simulink model "nav21"  (R2020a)
settings: Solver=FixedStepDiscrete  StartTime=0.0  StopTime=inf  RelTol=1e-3
model workspace (MAT data in the model file):
  SL_ROS_VariableLengthArrays_MaxSizes.CommonInfo.ArrayTruncateAction = 'EmitWarning'
  SL_ROS_VariableLengthArrays_MaxSizes.MsgTypeMap = containers.Map
  SL_ROS_VariableLengthArrays_MaxSizes.MsgTypeMap.serialization.keys = {'nav_msgs/OccupancyGrid', 'sensor_msgs/CompressedImage', 'sensor_msgs/Image', 'std_msgs/Float64MultiArray'}
  SL_ROS_VariableLengthArrays_MaxSizes.MsgTypeMap.serialization.values{1}.PropertyName = 'Data'
  SL_ROS_VariableLengthArrays_MaxSizes.MsgTypeMap.serialization.values{1}.DataType = 'int8'
  SL_ROS_VariableLengthArrays_MaxSizes.MsgTypeMap.serialization.values{1}.MaxLength = 1000000
  SL_ROS_VariableLengthArrays_MaxSizes.MsgTypeMap.serialization.values{2}(1).PropertyName = 'Data'
  SL_ROS_VariableLengthArrays_MaxSizes.MsgTypeMap.serialization.values{2}(1).DataType = 'uint8'
  SL_ROS_VariableLengthArrays_MaxSizes.MsgTypeMap.serialization.values{2}(1).MaxLength = 36000
  SL_ROS_VariableLengthArrays_MaxSizes.MsgTypeMap.serialization.values{2}(2).PropertyName = 'Format'
  SL_ROS_VariableLengthArrays_MaxSizes.MsgTypeMap.serialization.values{2}(2).DataType = 'uint8'
  SL_ROS_VariableLengthArrays_MaxSizes.MsgTypeMap.serialization.values{2}(2).MaxLength = 128
  SL_ROS_VariableLengthArrays_MaxSizes.MsgTypeMap.serialization.values{3}(1).PropertyName = 'Data'
  SL_ROS_VariableLengthArrays_MaxSizes.MsgTypeMap.serialization.values{3}(1).DataType = 'uint8'
  SL_ROS_VariableLengthArrays_MaxSizes.MsgTypeMap.serialization.values{3}(1).MaxLength = 921600
  SL_ROS_VariableLengthArrays_MaxSizes.MsgTypeMap.serialization.values{3}(2).PropertyName = 'Encoding'
  SL_ROS_VariableLengthArrays_MaxSizes.MsgTypeMap.serialization.values{3}(2).DataType = 'uint8'
  SL_ROS_VariableLengthArrays_MaxSizes.MsgTypeMap.serialization.values{3}(2).MaxLength = 128
  SL_ROS_VariableLengthArrays_MaxSizes.MsgTypeMap.serialization.values{4}.PropertyName = 'Data'
  SL_ROS_VariableLengthArrays_MaxSizes.MsgTypeMap.serialization.values{4}.DataType = 'double'
  SL_ROS_VariableLengthArrays_MaxSizes.MsgTypeMap.serialization.values{4}.MaxLength = 32
  SL_ROS_VariableLengthArrays_MaxSizes.MsgTypeMap.serialization.uniformity = 0
  SL_ROS_VariableLengthArrays_MaxSizes.MsgTypeMap.serialization.keyType = 'char'
  SL_ROS_VariableLengthArrays_MaxSizes.MsgTypeMap.serialization.valueType = 'any'
values from neighbouring files (symbols this model uses):
  chargingStn = [setInitialPose(1,1), setInitialPose(1,2)]    [startup.m]
  L2RTransform = [cos(L2Rtheta), -sin(L2Rtheta), L2Rx ... (first row only)    [startup.m]
  LIVE_MODE = 1    [startup.m]
  map = binaryOccupancyMap(logicalMap, 1/0.05)    [exampleHelperVisualizeExecuteRobots.m]
  W2LOTransform = W2ORTransform/(L2RTransform)    [startup.m]
  W2ORtheta = setInitialPose(1,3)    [startup.m]
  waypoints = [-2.5, 0 ... (first row only)    [startup.m]
  wheelBase = 0.4464    [startup.m]
  wheelRadius = 0.1715/2    (= 0.08575)    [startup.m]
undefined symbols (not defined in the file or in its folder): Angular, Data, Data_SL_Info, gray, Linear, loadingStn, unloadingStn
libraries: robotlib x14, robotalgslib x3, simulink x2, vrlib x1
settings Model: EnablePacing=on  OrderedModelArguments=off  Creator=john  LastModifiedBy=john
settings OptimizationCC: EnhancedBackFolding=on  PassReuseOutputArgsAs=Individual arguments  ZeroExternalMemoryAtStartup=off  ZeroInternalMemoryAtStartup=off  MaxStackSize=64  OptimizeBlockOrder=speed  DifferentSizesBufferReuse=on  OptimizationCustomize=off  EfficientTunableParamExpr=on
settings DebuggingCC: ParameterTunabilityLossMsg=error
settings HardwareCC: ProdBitPerPointer=32  ProdBitPerSizeT=32  ProdBitPerPtrDiffT=32  ProdLargestAtomicFloat=None  ProdIntDivRoundTo=Undefined  ProdEndianess=Unspecified  ProdWordSize=32  ProdHWDeviceType=Generic->Unspecified (assume 32-bit Generic)  UseEmbeddedCoderFeatures=off
settings RTWCC: SystemTargetFile=ert.tlc  HardwareBoard=Robot Operating System (ROS)  TemplateMakefile=ert_default_tmf  Toolchain=Catkin  TargetLang=C++
settings CodeAppCC: ForceParamTrailComments=on  IgnoreCustomStorageClasses=off  OperatorAnnotations=on  SimulinkDataObjDesc=on  SFDataObjDesc=on  InsertBlockDesc=on
settings ERTTargetCC: SupportNonInlinedSFcns=on

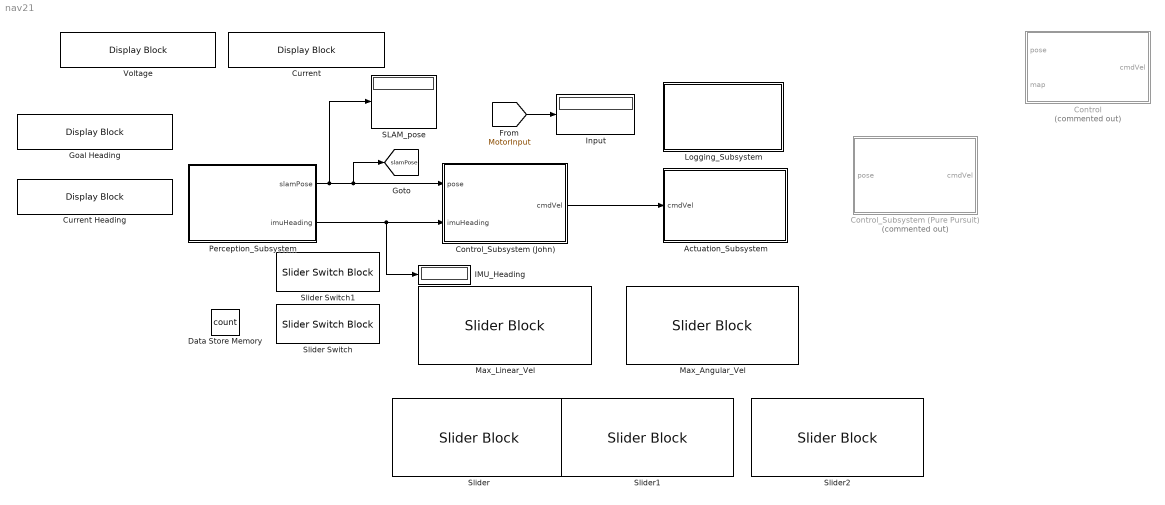
== system nav21 ==
  Actuation_Subsystem : Subsystem
  Control : Subsystem  Commented=on
  Control_Subsystem (John) : Subsystem
  Control_Subsystem (Pure Pursuit) : Subsystem  Commented=on
  Current : DisplayBlock  LabelPosition=Hide  Format=short  Transparency=1
  Current Heading : DisplayBlock  LabelPosition=Hide  Format=short  Transparency=1
  Data Store Memory : DataStoreMemory  DataStoreName=count  ReadBeforeWriteMsg=warning  WriteAfterWriteMsg=warning  WriteAfterReadMsg=warning  ShowAdditionalParam=off
  Goal Heading : DisplayBlock  LabelPosition=Hide  Format=short  Transparency=1
  IMU_Heading : Display
  Input : Display
  Logging_Subsystem : Subsystem
  Max_Angular_Vel : SliderBlock  ScaleMax=2
  Max_Linear_Vel : SliderBlock  ScaleMax=1.5
  Perception_Subsystem : Subsystem
  SLAM_pose : Display
  Slider : SliderBlock  ScaleMax=5
  Slider Switch : SliderSwitchBlock
      settings: Values={{'Off', 'On'}, [0 1]}
  Slider Switch1 : SliderSwitchBlock
      settings: Values={{'Off', 'On'}, [1 0]}
  Slider1 : SliderBlock  ScaleMax=1
  Slider2 : SliderBlock  ScaleMax=1.5
  Voltage : DisplayBlock  LabelPosition=Hide  Format=short  Transparency=1
  tag scope: slamPose=global
  wires:
  [MotorInput] -> Input/1
  Perception_Subsystem/2(imuHeading) -> IMU_Heading/1, Control_Subsystem (John)/2(imuHeading)
  Perception_Subsystem/1(slamPose) -> SLAM_pose/1, [slamPose], Control_Subsystem (John)/1(pose)
  Control_Subsystem (John)/1(cmdVel) -> Actuation_Subsystem/1(cmdVel)

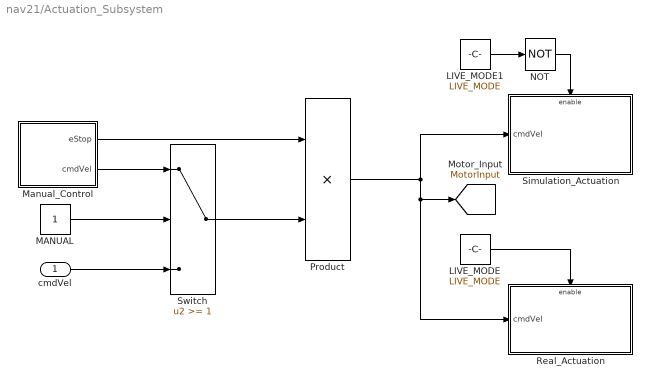
== system nav21/Actuation_Subsystem ==
  cmdVel : Inport
  LIVE_MODE : Constant  Value=LIVE_MODE
  LIVE_MODE1 : Constant  Value=LIVE_MODE
  MANUAL : Constant
  Manual_Control : Subsystem
  NOT : Logic  Operator=NOT  IconShape=distinctive  AllPortsSameDT=off  OutDataTypeStr=boolean
  Product : Product
  Real_Actuation : Subsystem
  Simulation_Actuation : Subsystem
  Switch : Switch  Threshold=1
  tag scope: MotorInput=global
  wires:
  cmdVel/1 -> Switch/3
  LIVE_MODE/1 -> Real_Actuation/Enable
  NOT/1 -> Simulation_Actuation/Enable
  LIVE_MODE1/1 -> NOT/1
  Switch/1 -> Product/2
  Product/1 -> [MotorInput], Real_Actuation/1(cmdVel), Simulation_Actuation/1(cmdVel)
  MANUAL/1 -> Switch/2
  Manual_Control/1(eStop) -> Product/1
  Manual_Control/2(cmdVel) -> Switch/1

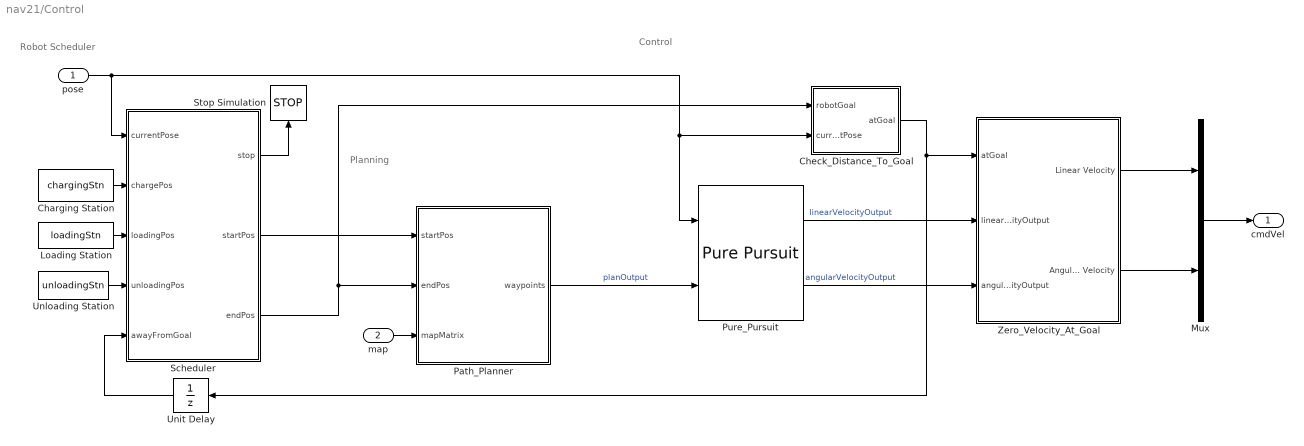
== system nav21/Control ==
  note: Control
  note: Robot Scheduler
  note: Planning
  pose : Inport
  map : Inport  Port=2
  "Charging Station " : Constant  Value=chargingStn  SampleTime=1
  Check_Distance_To_Goal : Subsystem
  Loading Station : Constant  Value=loadingStn
  Mux : Mux  Inputs=2
  Path_Planner : MATLAB Function  TreatAsAtomicUnit=on
  Pure_Pursuit : robotalgslib/Pure Pursuit  DesiredLinearVelocity=1  MaxAngularVelocity=0.5  LookaheadDistance=1  TargetDirPort=off  SimulateUsing=Code generation
  Scheduler : Stateflow chart  TreatAsAtomicUnit=on
  Stop Simulation : Stop
  Unit Delay : UnitDelay  SampleTime=-1  HasFrameUpgradeWarning=on
  Unloading Station : Constant  Value=unloadingStn  SampleTime=1
  Zero_Velocity_At_Goal : Subsystem
  cmdVel : Outport
  wires:
  Check_Distance_To_Goal/1(atGoal) -> Unit Delay/1, Zero_Velocity_At_Goal/1(atGoal)
  "Charging Station "/1 -> Scheduler/2(chargePos)
  Scheduler/2(startPos) -> Path_Planner/1(startPos)
  Unit Delay/1 -> Scheduler/5(awayFromGoal)
  Scheduler/3(endPos) -> Path_Planner/2(endPos), Check_Distance_To_Goal/1(robotGoal)
  Loading Station/1 -> Scheduler/3(loadingPos)
  Pure_Pursuit/2 -> Zero_Velocity_At_Goal/3(angularVelocityOutput)  "angularVelocityOutput"
  pose/1 -> Check_Distance_To_Goal/2(currentPose), Pure_Pursuit/1, Scheduler/1(currentPose)
  Unloading Station/1 -> Scheduler/4(unloadingPos)
  Scheduler/1(stop) -> Stop Simulation/1
  Path_Planner/1(waypoints) -> Pure_Pursuit/2  "planOutput"
  Pure_Pursuit/1 -> Zero_Velocity_At_Goal/2(linearVelocityOutput)  "linearVelocityOutput"
  Zero_Velocity_At_Goal/2(Angular Velocity) -> Mux/2
  Zero_Velocity_At_Goal/1(Linear Velocity) -> Mux/1
  Mux/1 -> cmdVel/1
  map/1 -> Path_Planner/3(mapMatrix)

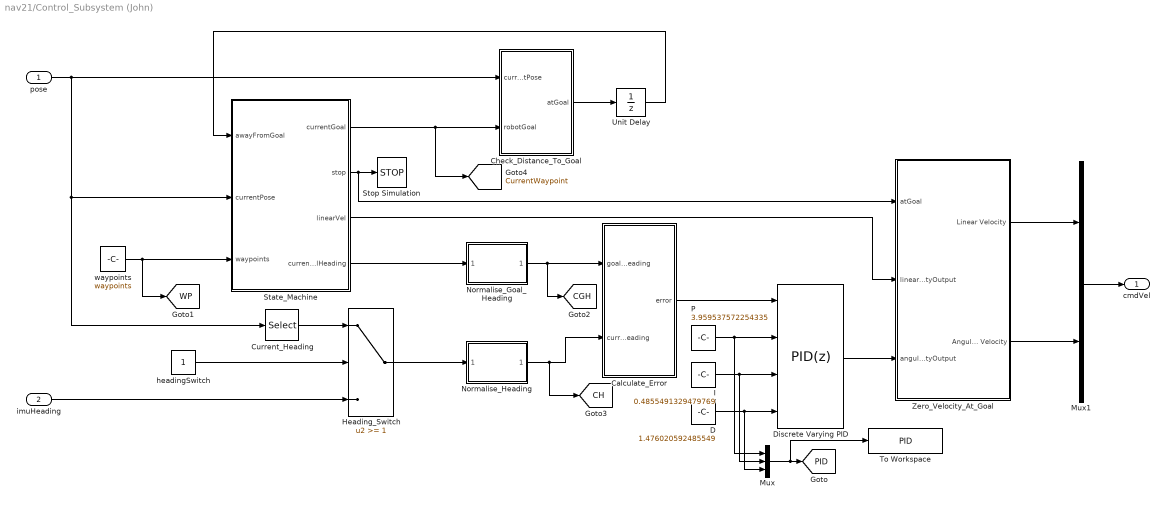
== system nav21/Control_Subsystem (John) ==
  pose : Inport
  imuHeading : Inport  Port=2
  Calculate_Error : MATLAB Function  TreatAsAtomicUnit=on
  Check_Distance_To_Goal : Subsystem
  Current_Heading : Selector  InputPortWidth=3  IndexOptions=Index vector (dialog)  Indices=[3]  OutputSizes=1
  D : Constant  Value=1.476020592485549
  Discrete Varying PID : simulink/Continuous/PID Controller  Controller=PID  Form=Parallel  TimeDomain=Discrete-time  UseExternalTs=off  SampleTime=-1  IntegratorMethod=Forward Euler  FilterMethod=Forward Euler  ControllerParametersSource=external  P=1  I=1  D=0  UseFilter=off  N=100  TunerSelectOption=Transfer Function Based (PID Tuner App)  InitialConditionSource=internal  InitialConditionForIntegrator=0  InitialConditionForFilter=0  DifferentiatorICPrevScaledInput=0  ExternalReset=none  TrackingMode=off  Kt=1  LimitOutput=on  UpperSaturationLimit=2  LowerSaturationLimit=-2  LinearizeAsGain=off  AntiWindupMode=clamping  Kb=1  POutMin=[]  POutMax=[]  IOutMin=[]  IOutMax=[]  DOutMin=[]  DOutMax=[]  NOutMin=[]  NOutMax=[]  SumOutMin=[]  SumOutMax=[]  SaturationOutMin=[]  SaturationOutMax=[]  PParamMin=[]  PParamMax=[]  IParamMin=[]  IParamMax=[]  DParamMin=[]  DParamMax=[]  NParamMin=[]  NParamMax=[]  KbParamMin=[]  KbParamMax=[]  KtParamMin=[]  KtParamMax=[]  KbOutMin=[]  KbOutMax=[]  KtOutMin=[]  KtOutMax=[]  IntegratorOutMin=[]  IntegratorOutMax=[]  FilterOutMin=[]  FilterOutMax=[]  SumI1OutMin=[]  SumI1OutMax=[]  SumI2OutMin=[]  SumI2OutMax=[]  SumI3OutMin=[]  SumI3OutMax=[]  SumI4OutMin=[]  SumI4OutMax=[]  SumDOutMin=[]  SumDOutMax=[]  DifferentiatorOutMin=[]  DifferentiatorOutMax=[]  FilterDiffOutCoefMin=[]  FilterDiffOutCoefMax=[]  ReciprocalOutMin=[]  ReciprocalOutMax=[]  SumDenOutMin=[]  SumDenOutMax=[]  SumNumOutMin=[]  SumNumOutMax=[]  DivideOutMin=[]  DivideOutMax=[]  UdiffTsProdOutMin=[]  UdiffTsProdOutMax=[]  NTsProdOutMin=[]  NTsProdOutMax=[]  UintegralTsProdOutMin=[]  UintegralTsProdOutMax=[]  UngainTsProdOutMin=[]  UngainTsProdOutMax=[]  IntegratorContinuousStateAttributes=''  IntegratorStateMustResolveToSignalObject=off  IntegratorRTWStateStorageClass=Auto  FilterContinuousStateAttributes=''  FilterStateMustResolveToSignalObject=off  FilterRTWStateStorageClass=Auto  ParallelPVariant=ExternalParameters  IdealPVariant=Disabled  IVariant=ExternalParameters  DVariant=ExternalParameters  IntegratorVariant=Discrete  SatVariant=Enabled  AWVariant=DiscClampingParallel  PCopyVariant=Disabled  TRVariant=Disabled  FdbkBlocksVariant=Forward  IdealPFdbkVariant=Disabled  SatFdbkVariant=Disabled  DerivativeFilterVariant=Differentiator  NVariant=Passthrough  NCopyVariant=Disabled_SignalSpec  FilterICVariant=InternalICsDifferentiator  IntegratorICVariant=InternalICs  ExternalResetVariant=Disabled  TRSumVariant=Passthrough  SumFdbkVariant=Disabled  SumVariant=Sum_PID  TsampFilterVariant=InternalTs  TsampNgainVariant=Passthrough  TsampIntegralVariant=Passthrough
  Heading_Switch : Switch  Threshold=1
  I : Constant  Value=0.4855491329479769
  Mux : Mux  Inputs=3
  Mux1 : Mux  Inputs=2
  Normalise_Goal_Heading : MATLAB Function  TreatAsAtomicUnit=on
  Normalise_Heading : MATLAB Function  TreatAsAtomicUnit=on
  P : Constant  Value=3.959537572254335
  State_Machine : Stateflow chart  TreatAsAtomicUnit=on
  Stop Simulation : Stop
  To Workspace : ToWorkspace  VariableName=PID  SaveFormat=Timeseries  SampleTime=-1
  Unit Delay : UnitDelay  SampleTime=-1  HasFrameUpgradeWarning=on
  Zero_Velocity_At_Goal : Subsystem
  headingSwitch : Constant  VectorParams1D=off
  waypoints : Constant  Value=waypoints  VectorParams1D=off
  cmdVel : Outport
  tag scope: CGH=global, CH=global, CurrentWaypoint=global, PID=global, WP=global
  wires:
  Mux1/1 -> cmdVel/1
  waypoints/1 -> State_Machine/3(waypoints), [WP]
  State_Machine/1(currentGoal) -> [CurrentWaypoint], Check_Distance_To_Goal/2(robotGoal)
  Unit Delay/1 -> State_Machine/1(awayFromGoal)
  Check_Distance_To_Goal/1(atGoal) -> Unit Delay/1
  State_Machine/2(stop) -> Zero_Velocity_At_Goal/1(atGoal), Stop Simulation/1
  pose/1 -> Current_Heading/1, State_Machine/2(currentPose), Check_Distance_To_Goal/1(currentPose)
  State_Machine/4(currentGoalHeading) -> Normalise_Goal_Heading/1(headingAngle)
  P/1 -> Discrete Varying PID/2, Mux/1
  D/1 -> Discrete Varying PID/4, Mux/3
  I/1 -> Mux/2, Discrete Varying PID/3
  Mux/1 -> To Workspace/1, [PID]
  Normalise_Heading/1(bearingAngle) -> [CH], Calculate_Error/2(currentHeading)
  Normalise_Goal_Heading/1(bearingAngle) -> [CGH], Calculate_Error/1(goalHeading)
  Calculate_Error/1(error) -> Discrete Varying PID/1
  Current_Heading/1 -> Heading_Switch/1
  Heading_Switch/1 -> Normalise_Heading/1(headingAngle)
  imuHeading/1 -> Heading_Switch/3
  headingSwitch/1 -> Heading_Switch/2
  Discrete Varying PID/1 -> Zero_Velocity_At_Goal/3(angularVelocityOutput)
  Zero_Velocity_At_Goal/2(Angular Velocity) -> Mux1/2
  Zero_Velocity_At_Goal/1(Linear Velocity) -> Mux1/1
  State_Machine/3(linearVel) -> Zero_Velocity_At_Goal/2(linearVelocityOutput)

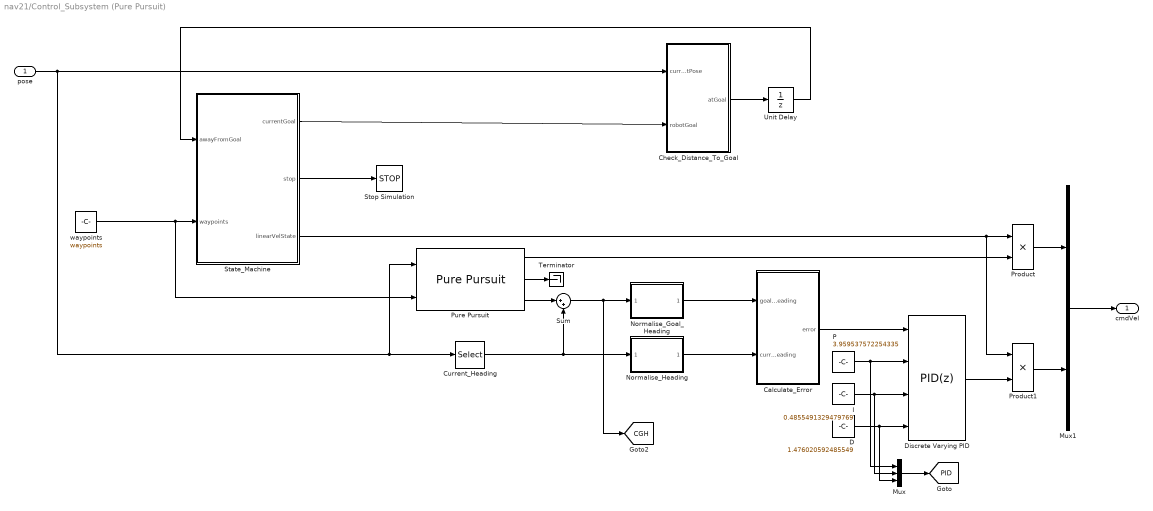
== system nav21/Control_Subsystem (Pure Pursuit) ==
  pose : Inport
  Calculate_Error : MATLAB Function  TreatAsAtomicUnit=on
  Check_Distance_To_Goal : Subsystem
  Current_Heading : Selector  InputPortWidth=3  IndexOptions=Index vector (dialog)  Indices=[3]  OutputSizes=1
  D : Constant  Value=1.476020592485549
  Discrete Varying PID : simulink/Continuous/PID Controller  Controller=PID  Form=Parallel  TimeDomain=Discrete-time  UseExternalTs=off  SampleTime=-1  IntegratorMethod=Forward Euler  FilterMethod=Forward Euler  ControllerParametersSource=external  P=1  I=1  D=0  UseFilter=off  N=100  TunerSelectOption=Transfer Function Based (PID Tuner App)  InitialConditionSource=internal  InitialConditionForIntegrator=0  InitialConditionForFilter=0  DifferentiatorICPrevScaledInput=0  ExternalReset=none  TrackingMode=off  Kt=1  LimitOutput=on  UpperSaturationLimit=2  LowerSaturationLimit=-2  LinearizeAsGain=off  AntiWindupMode=clamping  Kb=1  POutMin=[]  POutMax=[]  IOutMin=[]  IOutMax=[]  DOutMin=[]  DOutMax=[]  NOutMin=[]  NOutMax=[]  SumOutMin=[]  SumOutMax=[]  SaturationOutMin=[]  SaturationOutMax=[]  PParamMin=[]  PParamMax=[]  IParamMin=[]  IParamMax=[]  DParamMin=[]  DParamMax=[]  NParamMin=[]  NParamMax=[]  KbParamMin=[]  KbParamMax=[]  KtParamMin=[]  KtParamMax=[]  KbOutMin=[]  KbOutMax=[]  KtOutMin=[]  KtOutMax=[]  IntegratorOutMin=[]  IntegratorOutMax=[]  FilterOutMin=[]  FilterOutMax=[]  SumI1OutMin=[]  SumI1OutMax=[]  SumI2OutMin=[]  SumI2OutMax=[]  SumI3OutMin=[]  SumI3OutMax=[]  SumI4OutMin=[]  SumI4OutMax=[]  SumDOutMin=[]  SumDOutMax=[]  DifferentiatorOutMin=[]  DifferentiatorOutMax=[]  FilterDiffOutCoefMin=[]  FilterDiffOutCoefMax=[]  ReciprocalOutMin=[]  ReciprocalOutMax=[]  SumDenOutMin=[]  SumDenOutMax=[]  SumNumOutMin=[]  SumNumOutMax=[]  DivideOutMin=[]  DivideOutMax=[]  UdiffTsProdOutMin=[]  UdiffTsProdOutMax=[]  NTsProdOutMin=[]  NTsProdOutMax=[]  UintegralTsProdOutMin=[]  UintegralTsProdOutMax=[]  UngainTsProdOutMin=[]  UngainTsProdOutMax=[]  IntegratorContinuousStateAttributes=''  IntegratorStateMustResolveToSignalObject=off  IntegratorRTWStateStorageClass=Auto  FilterContinuousStateAttributes=''  FilterStateMustResolveToSignalObject=off  FilterRTWStateStorageClass=Auto  ParallelPVariant=ExternalParameters  IdealPVariant=Disabled  IVariant=ExternalParameters  DVariant=ExternalParameters  IntegratorVariant=Discrete  SatVariant=Enabled  AWVariant=DiscClampingParallel  PCopyVariant=Disabled  TRVariant=Disabled  FdbkBlocksVariant=Forward  IdealPFdbkVariant=Disabled  SatFdbkVariant=Disabled  DerivativeFilterVariant=Differentiator  NVariant=Passthrough  NCopyVariant=Disabled_SignalSpec  FilterICVariant=InternalICsDifferentiator  IntegratorICVariant=InternalICs  ExternalResetVariant=Disabled  TRSumVariant=Passthrough  SumFdbkVariant=Disabled  SumVariant=Sum_PID  TsampFilterVariant=InternalTs  TsampNgainVariant=Passthrough  TsampIntegralVariant=Passthrough
  I : Constant  Value=0.4855491329479769
  Mux : Mux  Inputs=3
  Mux1 : Mux  Inputs=2
  Normalise_Goal_Heading : MATLAB Function  TreatAsAtomicUnit=on
  Normalise_Heading : MATLAB Function  TreatAsAtomicUnit=on
  P : Constant  Value=3.959537572254335
  Product : Product
  Product1 : Product
  Pure Pursuit : robotalgslib/Pure Pursuit  DesiredLinearVelocity=0.1  MaxAngularVelocity=1.0  LookaheadDistance=lookAhead  TargetDirPort=on  SimulateUsing=Code generation
  State_Machine : Stateflow chart  TreatAsAtomicUnit=on
  Stop Simulation : Stop
  Sum : Sum  Inputs=|++
  Terminator : Terminator
  Unit Delay : UnitDelay  SampleTime=-1  HasFrameUpgradeWarning=on
  waypoints : Constant  Value=waypoints  VectorParams1D=off
  cmdVel : Outport
  tag scope: CGH=global, PID=global
  wires:
  Mux1/1 -> cmdVel/1
  waypoints/1 -> Pure Pursuit/2, State_Machine/2(waypoints)
  State_Machine/1(currentGoal) -> Check_Distance_To_Goal/2(robotGoal)
  Unit Delay/1 -> State_Machine/1(awayFromGoal)
  Check_Distance_To_Goal/1(atGoal) -> Unit Delay/1
  pose/1 -> Pure Pursuit/1, Current_Heading/1, Check_Distance_To_Goal/1(currentPose)
  P/1 -> Discrete Varying PID/2, Mux/1
  D/1 -> Discrete Varying PID/4, Mux/3
  I/1 -> Discrete Varying PID/3, Mux/2
  Mux/1 -> [PID]
  Current_Heading/1 -> Sum/2, Normalise_Heading/1(headingAngle)
  Normalise_Heading/1(bearingAngle) -> Calculate_Error/2(currentHeading)
  Normalise_Goal_Heading/1(bearingAngle) -> Calculate_Error/1(goalHeading)
  Calculate_Error/1(error) -> Discrete Varying PID/1
  Pure Pursuit/3 -> Sum/1
  Pure Pursuit/2 -> Terminator/1
  Pure Pursuit/1 -> Product/2
  Product/1 -> Mux1/1
  State_Machine/3(linearVelState) -> Product/1, Product1/1
  Discrete Varying PID/1 -> Product1/2
  Product1/1 -> Mux1/2
  State_Machine/2(stop) -> Stop Simulation/1
  Sum/1 -> [CGH], Normalise_Goal_Heading/1(headingAngle)

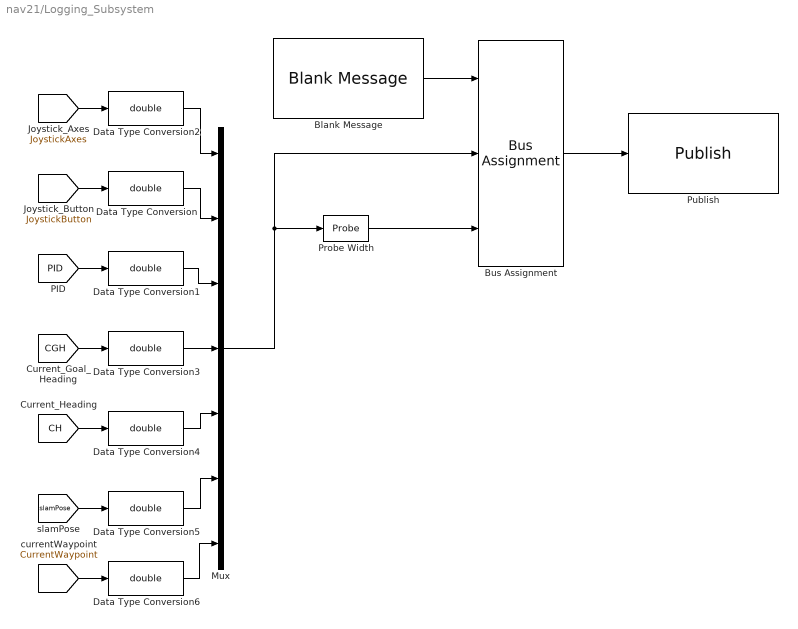
== system nav21/Logging_Subsystem ==
  Blank Message : robotlib/Blank Message  messageClass=Message  entityType=std_msgs/Float64MultiArray  messageType=std_msgs/Float64MultiArray  SampleTime=inf
  Bus Assignment : BusAssignment  AssignedSignals=Data,Data_SL_Info.CurrentLength
  Data Type Conversion{,1..6} (7 alike) : DataTypeConversion  OutDataTypeStr=double
  Mux : Mux  Inputs=7
  Probe Width : Probe  ProbeSampleTime=off  ProbeComplexSignal=off  ProbeWidthDataType=uint32
  Publish : robotlib/Publish  topicSource=Specify your own  topic=/amr/log  messageType=std_msgs/Float64MultiArray  messageQueueLength=1
  wires:
  [JoystickButton] -> Data Type Conversion/1
  [JoystickAxes] -> Data Type Conversion2/1
  Blank Message/1 -> Bus Assignment/1
  Bus Assignment/1 -> Publish/1
  Probe Width/1 -> Bus Assignment/3
  Mux/1 -> Bus Assignment/2, Probe Width/1
  Data Type Conversion/1 -> Mux/2
  [PID] -> Data Type Conversion1/1
  Data Type Conversion1/1 -> Mux/3
  Data Type Conversion2/1 -> Mux/1
  [CGH] -> Data Type Conversion3/1
  Data Type Conversion3/1 -> Mux/4
  [CH] -> Data Type Conversion4/1
  Data Type Conversion4/1 -> Mux/5
  [slamPose] -> Data Type Conversion5/1
  Data Type Conversion5/1 -> Mux/6
  [CurrentWaypoint] -> Data Type Conversion6/1
  Data Type Conversion6/1 -> Mux/7

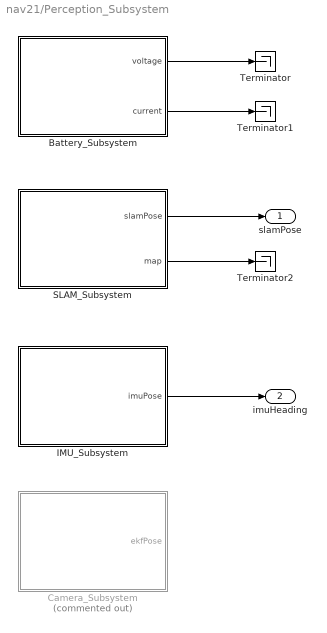
== system nav21/Perception_Subsystem ==
  Battery_Subsystem : Subsystem
  Camera_Subsystem : Subsystem  Commented=on
  IMU_Subsystem : Subsystem
  SLAM_Subsystem : Subsystem
  Terminator : Terminator
  Terminator1 : Terminator
  Terminator2 : Terminator
  slamPose : Outport
  imuHeading : Outport  Port=2
  wires:
  SLAM_Subsystem/1(slamPose) -> slamPose/1
  Battery_Subsystem/1(voltage) -> Terminator/1
  Battery_Subsystem/2(current) -> Terminator1/1
  SLAM_Subsystem/2(map) -> Terminator2/1
  IMU_Subsystem/1(imuPose) -> imuHeading/1

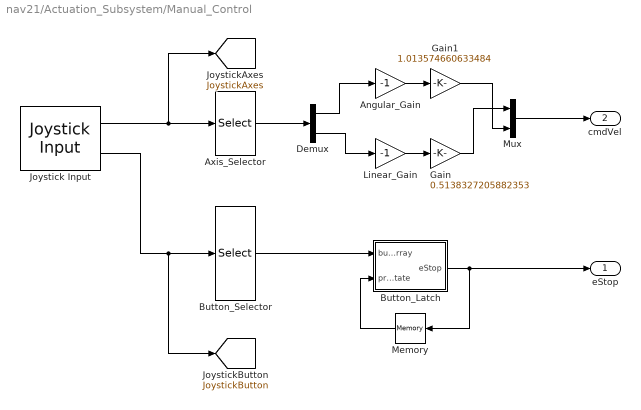
== system nav21/Actuation_Subsystem/Manual_Control ==
  Angular_Gain : Gain  Gain=-1
  Axis_Selector : Selector  InputPortWidth=8  IndexOptions=Index vector (dialog)  Indices=[1 2]  OutputSizes=1
  Button_Latch : MATLAB Function  TreatAsAtomicUnit=on
  Button_Selector : Selector  InputPortWidth=13  IndexOptions=Index vector (dialog)  Indices=[1 3]  OutputSizes=1
  Demux : Demux  Outputs=2
  Gain : Gain  Gain=0.5138327205882353
  Gain1 : Gain  Gain=1.013574660633484
  Joystick Input : vrlib/Joystick Input  joyid=1  adjustports=on  forcefeed=off
  Linear_Gain : Gain  Gain=-1
  Memory : Memory  InitialCondition=1
  Mux : Mux  Inputs=2
  eStop : Outport
  cmdVel : Outport  Port=2
  tag scope: JoystickAxes=global, JoystickButton=global
  wires:
  Demux/1 -> Angular_Gain/1
  Axis_Selector/1 -> Demux/1
  Demux/2 -> Linear_Gain/1
  Joystick Input/1 -> [JoystickAxes], Axis_Selector/1
  Mux/1 -> cmdVel/1
  Joystick Input/2 -> [JoystickButton], Button_Selector/1
  Memory/1 -> Button_Latch/2(prevEState)
  Button_Selector/1 -> Button_Latch/1(buttonArray)
  Button_Latch/1(eStop) -> eStop/1, Memory/1
  Linear_Gain/1 -> Gain/1
  Gain/1 -> Mux/1
  Angular_Gain/1 -> Gain1/1
  Gain1/1 -> Mux/2

== system nav21/Actuation_Subsystem/Real_Actuation ==
  cmdVel : Inport
  Enable : EnablePort
  Actuator : Subsystem
  Demux : Demux  Outputs=2
  Forward Kinematics : Subsystem
  wires:
  Forward Kinematics/1(leftRpmOut) -> Actuator/1(leftRPM)
  Demux/1 -> Forward Kinematics/1(v_in)
  Forward Kinematics/2(rightRpmOut) -> Actuator/2(rightRPM)
  Demux/2 -> Forward Kinematics/2(w_in)
  cmdVel/1 -> Demux/1

== system nav21/Actuation_Subsystem/Simulation_Actuation ==
  cmdVel : Inport
  Enable : EnablePort
  Blank Message : robotlib/Blank Message  messageClass=Message  entityType=geometry_msgs/Twist  messageType=geometry_msgs/Twist  SampleTime=inf
  Bus Assignment : BusAssignment  AssignedSignals=Linear.X,Angular.Z
  Demux : Demux  Outputs=2
  Publish : robotlib/Publish  topicSource=Select from ROS network  topic=/sim_cmd_vel  messageType=geometry_msgs/Twist  messageQueueLength=1
  wires:
  Blank Message/1 -> Bus Assignment/1
  Bus Assignment/1 -> Publish/1
  Demux/2 -> Bus Assignment/3
  Demux/1 -> Bus Assignment/2
  cmdVel/1 -> Demux/1

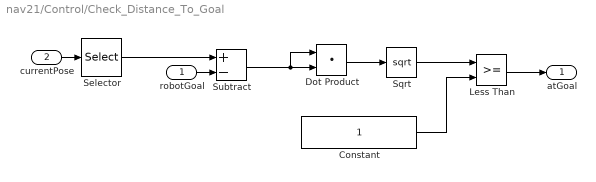
== system nav21/Control/Check_Distance_To_Goal ==
  robotGoal : Inport
  currentPose : Inport  Port=2
  Constant : Constant
  Dot Product : DotProduct  InputSameDT=on  OutDataTypeStr=Inherit: Inherit via internal rule
  Less Than : RelationalOperator  OutDataTypeStr=boolean  RndMeth=Simplest
  Selector : Selector  InputPortWidth=3  IndexOptions=Index vector (dialog)  Indices=[1 2]  OutputSizes=1
  Sqrt : Sqrt  SaturateOnIntegerOverflow=on
  Subtract : Sum  Inputs=+-
  atGoal : Outport
  wires:
  robotGoal/1 -> Subtract/2
  Dot Product/1 -> Sqrt/1
  Constant/1 -> Less Than/2
  currentPose/1 -> Selector/1
  Less Than/1 -> atGoal/1
  Sqrt/1 -> Less Than/1
  Subtract/1 -> Dot Product/1, Dot Product/2
  Selector/1 -> Subtract/1

== system nav21/Control/Zero_Velocity_At_Goal ==
  atGoal : Inport
  linearVelocityOutput : Inport  Port=2
  angularVelocityOutput : Inport  Port=3
  Product : Product
  Product1 : Product
  Linear Velocity : Outport  OutDataTypeStr=double
  Angular Velocity : Outport  Port=2  OutDataTypeStr=double
  wires:
  atGoal/1 -> Product1/1, Product/1
  angularVelocityOutput/1 -> Product1/2
  linearVelocityOutput/1 -> Product/2
  Product/1 -> Linear Velocity/1
  Product1/1 -> Angular Velocity/1

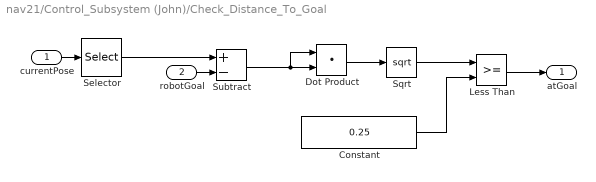
== system nav21/Control_Subsystem (John)/Check_Distance_To_Goal ==
  currentPose : Inport
  robotGoal : Inport  Port=2
  Constant : Constant  Value=0.25
  Dot Product : DotProduct  InputSameDT=on  OutDataTypeStr=Inherit: Inherit via internal rule
  Less Than : RelationalOperator  OutDataTypeStr=boolean  RndMeth=Simplest
  Selector : Selector  InputPortWidth=3  IndexOptions=Index vector (dialog)  Indices=[1 2]  OutputSizes=1
  Sqrt : Sqrt  SaturateOnIntegerOverflow=on
  Subtract : Sum  Inputs=+-
  atGoal : Outport
  wires:
  robotGoal/1 -> Subtract/2
  Dot Product/1 -> Sqrt/1
  Constant/1 -> Less Than/2
  currentPose/1 -> Selector/1
  Less Than/1 -> atGoal/1
  Sqrt/1 -> Less Than/1
  Subtract/1 -> Dot Product/1, Dot Product/2
  Selector/1 -> Subtract/1

== system nav21/Control_Subsystem (John)/State_Machine/CalculatePPHeading ==
  currentPose : Inport  OutDataTypeStr=double  PortDimensions=3
  startWaypoint : Inport  Port=2  OutDataTypeStr=double  PortDimensions=[1 2]
  endWaypoint : Inport  Port=3  OutDataTypeStr=double  PortDimensions=[1 2]
  f : TriggerPort  TriggerType=function-call  VariantControl=(inherit)
      settings: CopyFcn=Stateflow.SLINSF.SimulinkMan.removeBlockPreDeleteFcn  PreDeleteFcn=Stateflow.SLINSF.SimulinkMan.unsafePredeleteFcn
  Matrix Concatenate : Concatenate  Mode=Multidimensional array
  Pure Pursuit : robotalgslib/Pure Pursuit  DesiredLinearVelocity=0.1  MaxAngularVelocity=1.0  LookaheadDistance=1.0  TargetDirPort=on  SimulateUsing=Code generation
  Terminator : Terminator
  Terminator1 : Terminator
  heading : Outport
  wires:
  currentPose/1 -> Pure Pursuit/1
  Pure Pursuit/1 -> Terminator/1
  Pure Pursuit/2 -> Terminator1/1
  Pure Pursuit/3 -> heading/1
  endWaypoint/1 -> Matrix Concatenate/2
  startWaypoint/1 -> Matrix Concatenate/1
  Matrix Concatenate/1 -> Pure Pursuit/2

== system nav21/Control_Subsystem (John)/Zero_Velocity_At_Goal ==
  atGoal : Inport
  linearVelocityOutput : Inport  Port=2
  angularVelocityOutput : Inport  Port=3
  NOT : Logic  Operator=NOT  IconShape=distinctive  AllPortsSameDT=off  OutDataTypeStr=boolean
  Product : Product
  Product1 : Product
  Linear Velocity : Outport  OutDataTypeStr=double
  Angular Velocity : Outport  Port=2  OutDataTypeStr=double
  wires:
  angularVelocityOutput/1 -> Product1/2
  linearVelocityOutput/1 -> Product/2
  Product/1 -> Linear Velocity/1
  Product1/1 -> Angular Velocity/1
  atGoal/1 -> NOT/1
  NOT/1 -> Product/1, Product1/1

== system nav21/Control_Subsystem (Pure Pursuit)/Check_Distance_To_Goal ==
  currentPose : Inport
  robotGoal : Inport  Port=2
  Constant : Constant  Value=0.25
  Dot Product : DotProduct  InputSameDT=on  OutDataTypeStr=Inherit: Inherit via internal rule
  Less Than : RelationalOperator  OutDataTypeStr=boolean  RndMeth=Simplest
  Selector : Selector  InputPortWidth=3  IndexOptions=Index vector (dialog)  Indices=[1 2]  OutputSizes=1
  Sqrt : Sqrt  SaturateOnIntegerOverflow=on
  Subtract : Sum  Inputs=+-
  atGoal : Outport
  wires:
  robotGoal/1 -> Subtract/2
  Dot Product/1 -> Sqrt/1
  Constant/1 -> Less Than/2
  currentPose/1 -> Selector/1
  Less Than/1 -> atGoal/1
  Sqrt/1 -> Less Than/1
  Subtract/1 -> Dot Product/1, Dot Product/2
  Selector/1 -> Subtract/1

== system nav21/Perception_Subsystem/Battery_Subsystem ==
  Bus Selector : BusSelector  OutputSignals=Data
  Bus Selector1 : BusSelector  OutputSignals=Data
  Live_Subscriber : robotlib/Subscribe  topicSource=Select from ROS network  topic=/amr/status/voltage  messageType=std_msgs/Float32  sampleTime=-1  messageQueueLength=1
  Live_Subscriber1 : robotlib/Subscribe  topicSource=Select from ROS network  topic=/amr/status/current  messageType=std_msgs/Float32  sampleTime=-1  messageQueueLength=1
  Terminator : Terminator
  Terminator1 : Terminator
  voltage : Outport
  current : Outport  Port=2
  wires:
  Live_Subscriber/1 -> Terminator/1
  Live_Subscriber1/1 -> Terminator1/1
  Live_Subscriber/2 -> Bus Selector/1
  Live_Subscriber1/2 -> Bus Selector1/1
  Bus Selector/1 -> voltage/1  "<Data>"
  Bus Selector1/1 -> current/1  "<Data>"

== system nav21/Perception_Subsystem/Camera_Subsystem ==
  Live_Subscriber : robotlib/Subscribe  topicSource=Select from ROS network  topic=/zed_node/left_raw/image_raw_color/compressed  messageType=sensor_msgs/CompressedImage  sampleTime=-1  messageQueueLength=1
  MATLAB Function : MATLAB Function  TreatAsAtomicUnit=on
  Read Image : robotlib/Read Image  MaximumImageSize=[360, 640]  ImageEncoding=bgra8  ShowAlphaOutput=off  ShowErrorCodeOutput=off  VariableSizeOutputs=off
      settings: SourceProductBaseCode=RR
  Video Viewer : VideoViewer  FigPos=[741 936 701 539]
  ekfPose : Outport
  wires:
  Live_Subscriber/2 -> Read Image/1
  Read Image/1 -> MATLAB Function/1(image), Video Viewer/1
  MATLAB Function/1(y) -> ekfPose/1

== system nav21/Perception_Subsystem/IMU_Subsystem ==
  Live_Pose_Parser : Subsystem
  Live_Subscriber : robotlib/Subscribe  topicSource=Select from ROS network  topic=/tinkerforge_imu_ros/imu  messageType=sensor_msgs/Imu  sampleTime=-1  messageQueueLength=1
  Terminator : Terminator
  imuPose : Outport
  wires:
  Live_Subscriber/2 -> Live_Pose_Parser/1(msg)
  Live_Subscriber/1 -> Terminator/1
  Live_Pose_Parser/1(imuPose) -> imuPose/1

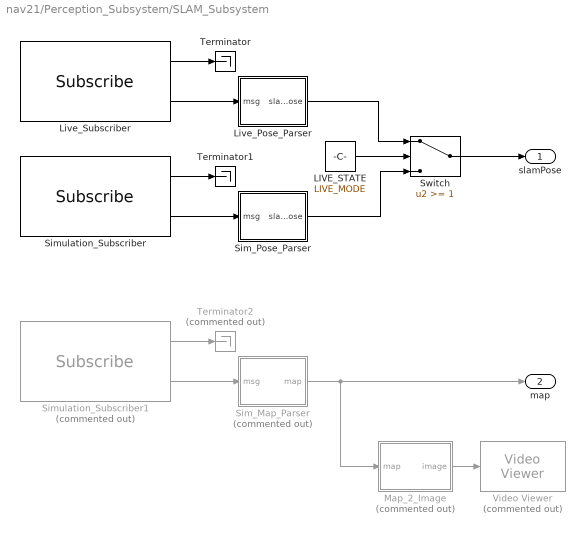
== system nav21/Perception_Subsystem/SLAM_Subsystem ==
  LIVE_STATE : Constant  Value=LIVE_MODE
  Live_Pose_Parser : Subsystem
  Live_Subscriber : robotlib/Subscribe  topicSource=Select from ROS network  topic=/slamware_ros_sdk_server_node/odom  messageType=nav_msgs/Odometry  sampleTime=-1  messageQueueLength=1
  Map_2_Image : MATLAB Function  Commented=on  TreatAsAtomicUnit=on
  Sim_Map_Parser : Subsystem  Commented=on
  Sim_Pose_Parser : Subsystem
  Simulation_Subscriber : robotlib/Subscribe  topicSource=Select from ROS network  topic=/amcl_pose  messageType=geometry_msgs/PoseWithCovarianceStamped  sampleTime=-1  messageQueueLength=1
  Simulation_Subscriber1 : robotlib/Subscribe  Commented=on  topicSource=Select from ROS network  topic=/map  messageType=nav_msgs/OccupancyGrid  sampleTime=-1  messageQueueLength=1
  Switch : Switch  Threshold=1
  Terminator : Terminator
  Terminator1 : Terminator
  Terminator2 : Terminator  Commented=on
  Video Viewer : VideoViewer  Commented=on  colormapValue=gray(256)  FigPos=[1099 872 703 501]
  slamPose : Outport
  map : Outport  Port=2
  wires:
  LIVE_STATE/1 -> Switch/2
  Live_Subscriber/2 -> Live_Pose_Parser/1(msg)
  Simulation_Subscriber/2 -> Sim_Pose_Parser/1(msg)
  Sim_Pose_Parser/1(slamPose) -> Switch/3
  Live_Pose_Parser/1(slamPose) -> Switch/1
  Switch/1 -> slamPose/1
  Simulation_Subscriber/1 -> Terminator1/1
  Live_Subscriber/1 -> Terminator/1
  Simulation_Subscriber1/2 -> Sim_Map_Parser/1(msg)
  Sim_Map_Parser/1(map) -> map/1, Map_2_Image/1(map)
  Map_2_Image/1(image) -> Video Viewer/1
  Simulation_Subscriber1/1 -> Terminator2/1

== system nav21/Actuation_Subsystem/Real_Actuation/Actuator ==
  leftRPM : Inport
  rightRPM : Inport  Port=2
  Blank Message : robotlib/Blank Message  messageClass=Message  entityType=geometry_msgs/Twist  messageType=geometry_msgs/Twist  SampleTime=inf
  Bus Assignment : BusAssignment  AssignedSignals=Angular.X,Angular.Y
  Publish : robotlib/Publish  topicSource=Select from ROS network  topic=/zlac8015d/rpm  messageType=geometry_msgs/Twist  messageQueueLength=1
  wires:
  Bus Assignment/1 -> Publish/1
  Blank Message/1 -> Bus Assignment/1
  rightRPM/1 -> Bus Assignment/3
  leftRPM/1 -> Bus Assignment/2

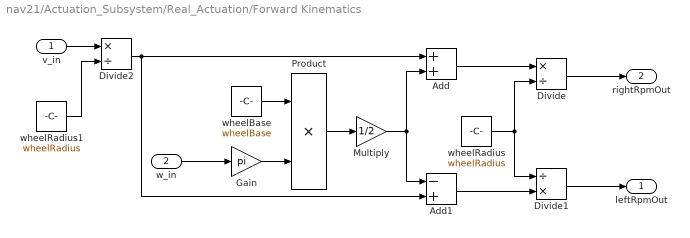
== system nav21/Actuation_Subsystem/Real_Actuation/Forward Kinematics ==
  v_in : Inport
  w_in : Inport  Port=2
  Add : Sum
  Add1 : Sum  Inputs=-+
  Divide : Product  Inputs=*/
  Divide1 : Product  Inputs=/*
  Divide2 : Product  Inputs=*/
  Gain : Gain  Gain=pi
  Multiply : Gain  Gain=1/2
  Product : Product
  wheelBase : Constant  Value=wheelBase
  wheelRadius : Constant  Value=wheelRadius
  wheelRadius1 : Constant  Value=wheelRadius
  leftRpmOut : Outport
  rightRpmOut : Outport  Port=2
  wires:
  wheelBase/1 -> Product/1
  Product/1 -> Multiply/1
  Multiply/1 -> Add/2, Add1/1
  Add1/1 -> Divide1/2
  Add/1 -> Divide/1
  wheelRadius/1 -> Divide1/1, Divide/2
  Divide1/1 -> leftRpmOut/1
  Divide/1 -> rightRpmOut/1
  v_in/1 -> Divide2/1
  Divide2/1 -> Add/1, Add1/2
  wheelRadius1/1 -> Divide2/2
  Gain/1 -> Product/2
  w_in/1 -> Gain/1

== system nav21/Perception_Subsystem/IMU_Subsystem/Live_Pose_Parser ==
  msg : Inport
  Bus Selector2 : BusSelector  OutputSignals=Orientation.X,Orientation.Y,Orientation.Z,Orientation.W
  Coordinate_Transform : Sum
  Quaternion_2_Euler : MATLAB Function  TreatAsAtomicUnit=on
  W2RTheta : Constant  Value=W2ORtheta
  imuPose : Outport
  wires:
  msg/1 -> Bus Selector2/1
  Bus Selector2/4 -> Quaternion_2_Euler/4(w)  "<W>"
  Bus Selector2/3 -> Quaternion_2_Euler/3(z)  "<Z>"
  Bus Selector2/2 -> Quaternion_2_Euler/2(y)  "<Y>"
  Bus Selector2/1 -> Quaternion_2_Euler/1(x)  "<X>"
  Quaternion_2_Euler/1(theta) -> Coordinate_Transform/1
  Coordinate_Transform/1 -> imuPose/1
  W2RTheta/1 -> Coordinate_Transform/2

== system nav21/Perception_Subsystem/SLAM_Subsystem/Live_Pose_Parser ==
  msg : Inport
  Bus Selector2 : BusSelector  OutputSignals=Pose.Pose.Position.X,Pose.Pose.Position.Y,Pose.Pose.Orientation.X,Pose.Pose.Orientation.Y,Pose.Pose.Orientation.Z,Pose.Pose.Orientation.W
  L2R : Constant  Value=L2RTransform
  Mux : Mux  Inputs=3
  Quaternion_2_Euler : MATLAB Function  TreatAsAtomicUnit=on
  W2OL : Constant  Value=W2LOTransform
  World to Robot Transform : MATLAB Function  TreatAsAtomicUnit=on
  slamPose : Outport
  wires:
  msg/1 -> Bus Selector2/1
  Bus Selector2/1 -> Mux/1  "<X>"
  Bus Selector2/2 -> Mux/2  "<Y>"
  Bus Selector2/3 -> Quaternion_2_Euler/1(x)  "<X>"
  Bus Selector2/4 -> Quaternion_2_Euler/2(y)  "<Y>"
  Bus Selector2/5 -> Quaternion_2_Euler/3(z)  "<Z>"
  Bus Selector2/6 -> Quaternion_2_Euler/4(w)  "<W>"
  Quaternion_2_Euler/1(theta) -> Mux/3
  W2OL/1 -> World to Robot Transform/2(W2OLTransform)
  L2R/1 -> World to Robot Transform/3(L2RTransform)
  Mux/1 -> World to Robot Transform/1(pose)
  World to Robot Transform/1(robotPose) -> slamPose/1

== system nav21/Perception_Subsystem/SLAM_Subsystem/Sim_Map_Parser ==
  msg : Inport
  Bus Selector2 : BusSelector  OutputSignals=Data,Info.Width,Info.Height
  Map_Parser : MATLAB Function  TreatAsAtomicUnit=on
  map : Outport
  wires:
  msg/1 -> Bus Selector2/1
  Bus Selector2/1 -> Map_Parser/1(mapArray)  "<Data>"
  Map_Parser/1(logicalMatrix) -> map/1
  Bus Selector2/2 -> Map_Parser/2(mapWidth)  "<Width>"
  Bus Selector2/3 -> Map_Parser/3(mapHeight)  "<Height>"

== system nav21/Perception_Subsystem/SLAM_Subsystem/Sim_Pose_Parser ==
  msg : Inport
  Bus Selector2 : BusSelector  OutputSignals=Pose.Pose.Position.X,Pose.Pose.Position.Y,Pose.Pose.Orientation.X,Pose.Pose.Orientation.Y,Pose.Pose.Orientation.Z,Pose.Pose.Orientation.W
  Mux : Mux  Inputs=3
  Quaternion_2_Euler : MATLAB Function  TreatAsAtomicUnit=on
  slamPose : Outport
  wires:
  msg/1 -> Bus Selector2/1
  Mux/1 -> slamPose/1
  Bus Selector2/1 -> Mux/1  "<X>"
  Bus Selector2/2 -> Mux/2  "<Y>"
  Bus Selector2/3 -> Quaternion_2_Euler/1(x)  "<X>"
  Bus Selector2/4 -> Quaternion_2_Euler/2(y)  "<Y>"
  Bus Selector2/5 -> Quaternion_2_Euler/3(z)  "<Z>"
  Bus Selector2/6 -> Quaternion_2_Euler/4(w)  "<W>"
  Quaternion_2_Euler/1(theta) -> Mux/3

== matlab function nav21/Perception_Subsystem/SLAM_Subsystem/Sim_Pose_Parser/Quaternion_2_Euler ==
  data: x input; theta output; y input; z input; w input
function theta = fcn(x, y, z, w)

    euler = quat2eul([x, y, z, w]); 
    
    if sum(isnan(euler)) == 3
        
        euler = ([pi, 0, 0]);
        
    end 
    
theta = euler(1,3);

== matlab function nav21/Perception_Subsystem/SLAM_Subsystem/Sim_Map_Parser/Map_Parser ==
  data: mapArray input; logicalMatrix output size=[1000,1000]; mapWidth input; mapHeight input
function logicalMatrix = fcn(mapArray, mapWidth, mapHeight)

index = 1; 

% Check if width is larger then height
if mapWidth < mapHeight
    mapMatrix = zeros(mapHeight, 'int8'); 
else
    mapMatrix = zeros(mapWidth, 'int8'); 
end

% Remap 
for i = 1:mapHeight
    for j = 1:mapWidth 
        mapMatrix(i,j) = mapArray(index);
        index = index + 1; 
    end
end


logicalMatrix = imcomplement(mapMatrix < 100);

== matlab function nav21/Control/Path_Planner ==
  settings: updateMethod=DISCRETE
  data: startPos input size=[1 2]; endPos input size=[1 2]; waypoints output size=[500 2]; mapMatrix input
function waypoints = planning(startPos, endPos, mapMatrix)

persistent waypointsInternal
persistent prevStartPos
persistent prevEndPos

% Set constant parameters
maxNumNodes = 500;
robotLength = 0.775;

% Initialize persistent variables that are used downstream
if isempty(prevStartPos)
    prevStartPos = startPos;
end

if isempty(prevEndPos)
    prevEndPos = endPos;
end

isNewPath = (~isequal(prevStartPos, startPos) || ~isequal(prevEndPos, endPos));

if isempty(waypointsInternal) || isNewPath
    % Two conditions in which waypoints must be set: they are not yet
    % initialized, or they are initialized, but the current start and end
    % do not match those used to generate the previous set of waypoints
    [waypointsInternal] = planPath(mapMatrix, maxNumNodes, startPos, endPos);
end

% Update the outputs
waypoints = waypointsInternal;

% Update the persistent variables that indicate previous state
prevStartPos = startPos;
prevEndPos = endPos;

%% Helper Function

function wayPoints = planPath(mapMatrix, maxNodes, startPos, endPos)
    
    % Create a probabilistic roadmap
    map = binaryOccupancyMap(mapMatrix, 1/0.05);
    inflate(map, robotLength/2);
    prm = mobileRobotPRM(map, maxNodes);
    
    % Find a path between two points
    xy = findpath(prm, startPos(:)', endPos(:)');
    wayPoints = repmat(endPos(:)', maxNodes, 1);
    
    % Number of nodes that are actually used
    numNodes = length(xy);
    wayPoints(1:numNodes,:) = xy;    

end

end

== matlab function nav21/Perception_Subsystem/SLAM_Subsystem/Live_Pose_Parser/World to Robot Transform ==
  data: pose input; robotPose output; W2OLTransform input; L2RTransform input
function robotPose = fcn(pose, W2OLTransform, L2RTransform)
    
    % O2L Transform 
    OL2LTransform = [cos(pose(3,1)), -sin(pose(3,1)), pose(1,1);
                    sin(pose(3,1)), cos(pose(3,1)), pose(2,1);
                    0,              0,              1];

    % Calculate World to Robot
    W2RTransform = W2OLTransform*OL2LTransform*L2RTransform; 
    

    % Create 3D Rotation matrix
    rotm = [W2RTransform(1,1), W2RTransform(1,2), 0;
                      W2RTransform(2,1), W2RTransform(2,2), 0; 
                      0                , 0                , 1;]; 
    
    % Extract axis angle
    quat = rotm2quat(rotm);
    heading = quat2eul(quat); 
    
robotPose = [W2RTransform(1,3); W2RTransform(2,3); heading(1,1)];

== matlab function nav21/Perception_Subsystem/SLAM_Subsystem/Map_2_Image ==
  data: map input; image output size=[1000,1000]
function image = fcn(map)

image = imcomplement(flipud(map));

== matlab function nav21/Perception_Subsystem/IMU_Subsystem/Live_Pose_Parser/Quaternion_2_Euler ==
  data: x input; theta output; y input; z input; w input
function theta = fcn(x, y, z, w)

    euler = quat2eul([x, y, z, w]); 
    
    if sum(isnan(euler)) == 3
        
        euler = ([pi, 0, 0]);
        
    end 
    
theta = euler(1,3);

== matlab function nav21/Actuation_Subsystem/Manual_Control/Button_Latch ==
  data: buttonArray input; prevEState input; eStop output size=1
function eStop = fcn(buttonArray, prevEState)

    % Copy previous E State
    currentEState = prevEState; 

    % Map Button Array
    eStopButton = buttonArray(1,1); 
    resetStopButton = buttonArray(2,1); 

    % Check if emergency button is pressed and st
    if eStopButton == 1
        
        % Set stop state to be 0
        currentEState = 0;
        
    % Check if reset button is pressed
    elseif resetStopButton == 1
        
        % Set stop state to be 0 
        currentEState = 1; 
        
    end

eStop = currentEState;

== matlab function nav21/Perception_Subsystem/SLAM_Subsystem/Live_Pose_Parser/Quaternion_2_Euler ==
  data: x input; theta output; y input; z input; w input
function theta = fcn(x, y, z, w)

    euler = quat2eul([x, y, z, w]); 
    
    if sum(isnan(euler)) == 3
        
        euler = ([pi, 0, 0]);
        
    end 
    
theta = euler(1,3);

== matlab function nav21/Control_Subsystem (Pure Pursuit)/Calculate_Error ==
  data: goalHeading input; currentHeading input; error output
function error = fcn(goalHeading, currentHeading)
    
    % Calculate basic error
    error = goalHeading - currentHeading;
    
    % Calculate angle wrap
    if error < -pi
        error = error + 2*pi;
    elseif error > pi
        error = (error - 2*pi);
    end

== matlab function nav21/Control_Subsystem (Pure Pursuit)/Normalise_Goal_Heading ==
  data: headingAngle input; bearingAngle output
function bearingAngle = fcn(headingAngle)
 
    if headingAngle < 0
        headingAngle = pi + (pi - abs(headingAngle)); 
    end

bearingAngle = headingAngle;

== stateflow chart nav21/Control/Scheduler ==
  settings: sampleTime=0.01
  state Unloading
    entry, during:
    endPos = unloadingPos';
  state Loading
    entry,during:
    endPos = loadingPos';
  state Charging
    entry, during:
    endPos = chargePos';
  (default) -> Loading : {startPos = chargePos';}
  Loading -> Unloading : [~awayFromGoal && after(stopDelay, tick)]
      |
      | {startPos = currentPose(1:2)';}
  Unloading -> Charging : [~awayFromGoal  && after(stopDelay, tick)]
      | {startPos = currentPose(1:2)';}
  Charging -> (junction 201) : [~awayFromGoal]{stop = 1;}
  data: currentPose input; stop output =0; chargePos input size=[2 1]; loadingPos input size=[2 1]; unloadingPos input size=[2 1]; startPos output size=[1, 2]; endPos output size=[1, 2]; awayFromGoal input; stopDelay local =5

== matlab function nav21/Perception_Subsystem/Camera_Subsystem/MATLAB Function ==
  data: image input; y output
function y = fcn(image)
    
    tagFamily = ['tag36h11']; 
    
    [id,loc,detectedFamily] = readAprilTag(image,tagFamily);
    
y = I;

== stateflow chart nav21/Control_Subsystem (John)/State_Machine ==
  state RotateToWaypoint
    entry:
    linearVel = 0;
    currentGoal = waypoints(count,:);
    currentGoalHeading = CalculateHeading(currentPose, currentGoal);
    during:
  state MoveToWaypoint
    entry:
    linearVel = 0.3;
    during:
    currentGoalHeading = CalculateHeading(currentPose, currentGoal);
    % currentGoalHeading = CalculatePPHeading(currentPose, waypoints(count,:), waypoints(count+1,:))
  state RotateToentry_
    linearVel = 0.0;
    currentGoal = waypoints(1,:);
    during:
    currentGoalHeading = CalculateHeading(currentPose, currentGoal);
    % currentGoalHeading = CalculatePPHeading(currentPose, waypoints(count,:), waypoints(count+1,:))
  state MoveToWaypoint2
    entry:
    linearVel = -0.3;
    currentGoal = waypoints(count,:);
    during:
    currentGoalHeading = CalculateReverseHeading(currentPose, currentGoal);
    %currentGoalHeading = CalculatePPHeading(currentPose, waypoints(count,:), waypoints(count+1,:))
    exit:
  state heading = CalculatePPHeading(currentPose,startWaypoint,endWaypoint) [function]
  (default) -> RotateToWaypoint : {count = 1;
      | [max,~] = size(waypoints);}
  RotateToWaypoint -> MoveToWaypoint : [currentGoalHeading - 0.05< currentPose(3) && currentPose(3) < currentGoalHeading + 0.05]
  MoveToWaypoint -> RotateToWaypoint [order 1] : [~awayFromGoal && count < max]
      | {count = count+1;}
  MoveToWaypoint -> RotateToentry_ [order 2] : [~awayFromGoal && count == max]
  MoveToWaypoint2 -> (junction 21) : [~awayFromGoal]
      | {stop = 1;}
  data: startPose function_input; endPose function_input; heading function_output; startPose function_input; endPose function_input; heading function_output; currentPose function_input double size=3; startWaypoint function_input double size=[1 2]; endWaypoint function_input double size=[1 2]; heading function_output; awayFromGoal input; currentGoal output; stop output; currentPose input; waypoints input; linearVel output; count local double; max local; currentGoalHeading output double
  function heading = CalculateHeading(startPose, endPose):
    | function heading = CalculateHeading(startPose, endPose)
    |    
    |    heading = atan2((endPose(1,2) - startPose(2,1)),(endPose(1,1) - startPose(1,1))); 
    |   
    | end
  function heading = CalculateReverseHeading(startPose, endPose):
    | function heading = CalculateReverseHeading(startPose, endPose)
    |    
    |    heading = atan2((startPose(2,1) - endPose(1,2)),(startPose(1,1) - endPose(1,1))); 
    |   
    | end

== matlab function nav21/Control_Subsystem (Pure Pursuit)/Normalise_Heading ==
  data: headingAngle input; bearingAngle output
function bearingAngle = fcn(headingAngle)
 
    if headingAngle < 0
        headingAngle = pi + (pi - abs(headingAngle)); 
    end

bearingAngle = headingAngle;

== matlab function nav21/Control_Subsystem (John)/Calculate_Error ==
  data: goalHeading input; currentHeading input; error output
function error = fcn(goalHeading, currentHeading)
    
    % Calculate basic error
    error = goalHeading - currentHeading;
    
    % Calculate angle wrap
    if error < -pi
        error = error + 2*pi;
    elseif error > pi
        error = (error - 2*pi);
    end

== matlab function nav21/Control_Subsystem (John)/Normalise_Heading ==
  data: headingAngle input; bearingAngle output
function bearingAngle = fcn(headingAngle)
 
    if headingAngle < 0
        headingAngle = pi + (pi - abs(headingAngle)); 
    end

bearingAngle = headingAngle;

== matlab function nav21/Control_Subsystem (John)/Normalise_Goal_Heading ==
  data: headingAngle input; bearingAngle output
function bearingAngle = fcn(headingAngle)
 
    if headingAngle < 0
        headingAngle = pi + (pi - abs(headingAngle)); 
    end

bearingAngle = headingAngle;

== stateflow chart nav21/Control_Subsystem (Pure Pursuit)/State_Machine ==
  state MoveToWaypoint
    entry:
    currentGoal = waypoints(max,:);
    during:
    linearVelState = 1;
    exit:
    linearVelState = 0;
  (default) -> MoveToWaypoint : {[max,~] = size(waypoints);}
  MoveToWaypoint -> (junction 21) : [~awayFromGoal]
      | {stop = 0;}
  data: awayFromGoal input; currentGoal output; stop output; waypoints input; max local; linearVelState output
